simulink model "sim005"  (R2023b)
settings: Solver=FixedStepAuto  StartTime=0.0  StopTime=10.0  FixedStep=0.001  RelTol=1e-3  EnableMultiTasking=on
values from neighbouring files (symbols this model uses):
  a1 = 40    [FK.m]    (also in IK_Analytical.m = 0.04; IK_MDH.m = 0.04; IK_Position.m = 0.04; IK_Solver.m = 0.04)
  a2 = 275    [FK.m]    (also in IK_Analytical.m = 0.275; IK_MDH.m = 0.275; IK_Position.m = 0.275; IK_Solver.m = 0.275)
  a3 = 25    [FK.m]    (also in IK_Analytical.m = 0.025; IK_MDH.m = 0.025; IK_Position.m = 0.025; IK_Solver.m = 0.025)
  d1 = 342    [FK.m]    (also in IK_Analytical.m = 0.342; IK_MDH.m = 0.342; IK_Position.m = 0.342; IK_Solver.m = 0.342)
  d4 = 280    [FK.m]    (also in IK_Analytical.m = 0.28; IK_MDH.m = 0.28; IK_Position.m = 0.28; IK_Solver.m = 0.28)
  fc1 = 0    [set_mode_parameter.m]
  fc2 = 0    [set_mode_parameter.m]
  fc3 = 0    [set_mode_parameter.m]
  fc4 = 0    [set_mode_parameter.m]
  fc5 = 0    [set_mode_parameter.m]
  fc6 = 0    [set_mode_parameter.m]
  fv1 = 0    [set_mode_parameter.m]
  fv2 = 0    [set_mode_parameter.m]
  fv3 = 0    [set_mode_parameter.m]
  fv4 = 0    [set_mode_parameter.m]
  fv5 = 0    [set_mode_parameter.m]
  fv6 = 0    [set_mode_parameter.m]
  Ia1 = 0    [set_mode_parameter.m]
  Ia2 = 0    [set_mode_parameter.m]
  Ia3 = 0    [set_mode_parameter.m]
  Ia4 = 0    [set_mode_parameter.m]
  Ia5 = 0    [set_mode_parameter.m]
  Ia6 = 0    [set_mode_parameter.m]
  Ic111 = 0    [set_mode_parameter.m]
  Ic112 = 0    [set_mode_parameter.m]
  Ic113 = 0    [set_mode_parameter.m]
  Ic122 = 0    [set_mode_parameter.m]
  Ic123 = 0    [set_mode_parameter.m]
  Ic133 = 1.3676    [set_mode_parameter.m]
  Ic211 = 8.8194    [set_mode_parameter.m]
  Ic212 = 0    [set_mode_parameter.m]
  Ic213 = 0    [set_mode_parameter.m]
  Ic222 = 6.0549    [set_mode_parameter.m]
  Ic223 = 0    [set_mode_parameter.m]
  Ic233 = 0.9569    [set_mode_parameter.m]
  Ic311 = 0.0332    [set_mode_parameter.m]
  Ic312 = 0    [set_mode_parameter.m]
  Ic313 = 0    [set_mode_parameter.m]
  Ic322 = 1.8442    [set_mode_parameter.m]
  Ic323 = 0    [set_mode_parameter.m]
  Ic333 = 1.0560    (= 1.056)    [set_mode_parameter.m]
  Ic411 = 0.1448    [set_mode_parameter.m]
  Ic412 = 0    [set_mode_parameter.m]
  Ic413 = 0    [set_mode_parameter.m]
  Ic422 = 0.0015    [set_mode_parameter.m]
  Ic423 = 0    [set_mode_parameter.m]
  Ic433 = 0.0822    [set_mode_parameter.m]
  Ic511 = 0    [set_mode_parameter.m]
  Ic512 = 0    [set_mode_parameter.m]
  Ic513 = 0    [set_mode_parameter.m]
  Ic522 = 0.0121    [set_mode_parameter.m]
  Ic523 = 0    [set_mode_parameter.m]
  Ic533 = 0.0299    [set_mode_parameter.m]
  Ic611 = 0.0134    [set_mode_parameter.m]
  Ic612 = 0    [set_mode_parameter.m]
  Ic613 = 0    [set_mode_parameter.m]
  Ic622 = 0    [set_mode_parameter.m]
  Ic623 = 0    [set_mode_parameter.m]
  Ic633 = 0.0051    [set_mode_parameter.m]
  m = (c1*px + s1*py) - dt*(c1*ax + s1*ay) - a1    [IK_6DOF_Robot.m]    (also in IK_MDH.m = pwx_1 - a1; IK_MDH_Robot.m = rho - a1)
  m1 = 0.167    [set_mode_parameter.m]
  m2 = 1    [set_mode_parameter.m]
  m3 = 0.5    [set_mode_parameter.m]
  m4 = 0.333    [set_mode_parameter.m]
  m5 = 0.25    [set_mode_parameter.m]
  m6 = 0.2    [set_mode_parameter.m]
  mc11 = 0    [set_mode_parameter.m]
  mc12 = 0    [set_mode_parameter.m]
  mc13 = 0.2    [set_mode_parameter.m]
  mc21 = 0.1291    [set_mode_parameter.m]
  mc22 = 0    [set_mode_parameter.m]
  mc23 = 3.3117    [set_mode_parameter.m]
  mc31 = 1.6484    [set_mode_parameter.m]
  mc32 = 0    [set_mode_parameter.m]
  mc33 = 0.8748    [set_mode_parameter.m]
  mc41 = 0.3200    (= 0.32)    [set_mode_parameter.m]
  mc42 = 0.2324    [set_mode_parameter.m]
  mc43 = 0.7083    [set_mode_parameter.m]
  mc51 = 0.4574    [set_mode_parameter.m]
  mc52 = 0    [set_mode_parameter.m]
  mc53 = 0.6427    [set_mode_parameter.m]
  mc61 = 0.3200    (= 0.32)    [set_mode_parameter.m]
  mc62 = -0.0513    [set_mode_parameter.m]
  mc63 = 0.6417    [set_mode_parameter.m]
  N = size(waypoints, 2)    [run_trajectory.m]
  s = zc - d(1)    [inverse_kinematics_6dof.m]
  XB4 = SerialLink([L1 L2 L3 L4 L5 L6], 'name', 'XB4')    [Toolbox_Motheds_1.m]
undefined symbols (not defined in the file or in its folder): X, Y, Z
libraries: sm_lib x56, nesl_utility x31, simulink x2
(part 2 of 2)

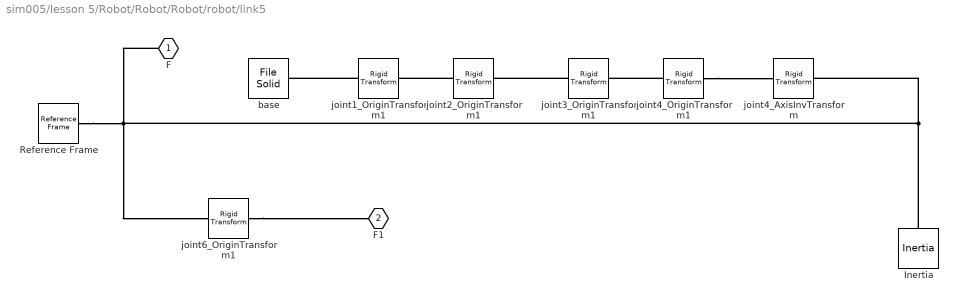
== system sim005/lesson 5/Robot/Robot/Robot/robot/link5 ==
  Inertia : sm_lib/Body Elements/Inertia  InertiaType=Custom  Mass=m5  MassUnits=kg  CenterOfMass=[mc51 mc52 mc53]  CenterOfMassUnits=m  MomentsOfInertia=[Ic511 Ic522 Ic533]  MomentsOfInertiaUnits=kg*m^2  ProductsOfInertia=[Ic523 Ic513 Ic512]  ProductsOfInertiaUnits=kg*m^2  GraphicType=Marker  MarkerShape=Inertia  MarkerSize=20  GraphicVisPropType=SimpleVisualProperties  GraphicDiffuseColor=[0.5 0.5 0.5]  GraphicSpecularColor=[0.5 0.5 0.5 1.0]  GraphicAmbientColor=[0.15 0.15 0.15 1.0]  GraphicEmissiveColor=[0.0 0.0 0.0 1.0]  GraphicShininess=75  GraphicOpacity=1.0
  Reference Frame : sm_lib/Frames and Transforms/Reference Frame
  base : sm_lib/Body Elements/File Solid  ExtGeomFileName=/home/jiehuang/Documents/Custom-Robot/Matlab_Study/Matlab2023Project/XB4-Robot/Mode/XB4-5.STL  UnitType=Custom  ExtGeomFileUnits=mm  StepReaderType=HEX  ExportConvexHullGeometry=off  InertiaType=Custom  Mass=0  MassUnits=kg  CenterOfMass=[0 0 0]  CenterOfMassUnits=m  MomentsOfInertia=[0 0 0]  MomentsOfInertiaUnits=kg*m^2  ProductsOfInertia=[0 0 0]  ProductsOfInertiaUnits=kg*m^2  BasedOnType=Density  Density=1000  DensityUnits=kg/(m^3)  DoExposeReferenceFrame=on  SerializedFrames=<Frames/>  GraphicType=FromGeometry  MarkerShape=Sphere  MarkerSize=10  GraphicVisPropType=SimpleVisualProperties  GraphicDiffuseColor=[0.5 0.5 0.5]  GraphicSpecularColor=[0.5 0.5 0.5 1.0]  GraphicAmbientColor=[0.15 0.15 0.15 1.0]  GraphicEmissiveColor=[0.0 0.0 0.0 1.0]  GraphicShininess=75  GraphicOpacity=1.0
  joint1_OriginTransform1 : sm_lib/Frames and Transforms/Rigid Transform  TranslationMethod=Cartesian  TranslationStandardOffset=0  TranslationStandardOffsetUnits=m  TranslationStandardAxis=+Z  TranslationCartesianOffset=[0 0 d1]  TranslationCartesianOffsetUnits=m  TranslationROffset=0  TranslationROffsetUnits=m  TranslationZOffset=0  TranslationZOffsetUnits=m  TranslationThetaOffset=0  TranslationThetaOffsetUnits=deg  RotationMethod=RotationSequence  RotationAngleUnits=deg  RotationStandardAxis=+Z  RotationAngle=0.0  RotationArbitraryAxis=[0 0 1]  FollAlignAxisA=+X  BaseAlignAxisA=+Y  FollAlignAxisB=+Y  BaseAlignAxisB=+Z  RotationSequenceAxes=BaseAxes  RotationSequence=XYZ  RotationSequenceAngles=[0 0 0]  RotationSequenceAnglesUnits=rad  RotationMatrix=[1 0 0; 0 1 0; 0 0 1]  Quaternion=[1 0 0 0]
  joint2_OriginTransform1 : sm_lib/Frames and Transforms/Rigid Transform  TranslationMethod=Cartesian  TranslationStandardOffset=0  TranslationStandardOffsetUnits=m  TranslationStandardAxis=+Z  TranslationCartesianOffset=[a1 0 0]  TranslationCartesianOffsetUnits=m  TranslationROffset=0  TranslationROffsetUnits=m  TranslationZOffset=0  TranslationZOffsetUnits=m  TranslationThetaOffset=0  TranslationThetaOffsetUnits=deg  RotationMethod=RotationSequence  RotationAngleUnits=deg  RotationStandardAxis=+Z  RotationAngle=0.0  RotationArbitraryAxis=[0 0 1]  FollAlignAxisA=+X  BaseAlignAxisA=+Y  FollAlignAxisB=+Y  BaseAlignAxisB=+Z  RotationSequenceAxes=FollowerAxes  RotationSequence=XYZ  RotationSequenceAngles=[-pi/2 0 -pi/2]  RotationSequenceAnglesUnits=rad  RotationMatrix=[1 0 0; 0 1 0; 0 0 1]  Quaternion=[1 0 0 0]
  joint3_OriginTransform1 : sm_lib/Frames and Transforms/Rigid Transform  TranslationMethod=Cartesian  TranslationStandardOffset=0  TranslationStandardOffsetUnits=m  TranslationStandardAxis=+Z  TranslationCartesianOffset=[a2 0 0]  TranslationCartesianOffsetUnits=m  TranslationROffset=0  TranslationROffsetUnits=m  TranslationZOffset=0  TranslationZOffsetUnits=m  TranslationThetaOffset=0  TranslationThetaOffsetUnits=deg  RotationMethod=RotationSequence  RotationAngleUnits=deg  RotationStandardAxis=+Z  RotationAngle=0.0  RotationArbitraryAxis=[0 0 1]  FollAlignAxisA=+X  BaseAlignAxisA=+Y  FollAlignAxisB=+Y  BaseAlignAxisB=+Z  RotationSequenceAxes=FollowerAxes  RotationSequence=XYZ  RotationSequenceAngles=[0 0 0]  RotationSequenceAnglesUnits=rad  RotationMatrix=[1 0 0; 0 1 0; 0 0 1]  Quaternion=[1 0 0 0]
  joint4_AxisInvTransform : sm_lib/Frames and Transforms/Rigid Transform  TranslationMethod=Cartesian  TranslationStandardOffset=0  TranslationStandardOffsetUnits=m  TranslationStandardAxis=+Z  TranslationCartesianOffset=[0 0 0]  TranslationCartesianOffsetUnits=m  TranslationROffset=0  TranslationROffsetUnits=m  TranslationZOffset=0  TranslationZOffsetUnits=m  TranslationThetaOffset=0  TranslationThetaOffsetUnits=deg  RotationMethod=RotationSequence  RotationAngleUnits=rad  RotationStandardAxis=+Z  RotationAngle=1.570796  RotationArbitraryAxis=[0 1 0]  FollAlignAxisA=+X  BaseAlignAxisA=+Y  FollAlignAxisB=+Y  BaseAlignAxisB=+Z  RotationSequenceAxes=FollowerAxes  RotationSequence=XYZ  RotationSequenceAngles=[pi/2 0 0]  RotationSequenceAnglesUnits=rad  RotationMatrix=[1 0 0; 0 1 0; 0 0 1]  Quaternion=[1 0 0 0]
  joint4_OriginTransform1 : sm_lib/Frames and Transforms/Rigid Transform  TranslationMethod=Cartesian  TranslationStandardOffset=0  TranslationStandardOffsetUnits=m  TranslationStandardAxis=+Z  TranslationCartesianOffset=[a3 d4 0]  TranslationCartesianOffsetUnits=m  TranslationROffset=0  TranslationROffsetUnits=m  TranslationZOffset=0  TranslationZOffsetUnits=m  TranslationThetaOffset=0  TranslationThetaOffsetUnits=deg  RotationMethod=RotationSequence  RotationAngleUnits=deg  RotationStandardAxis=+Z  RotationAngle=0.0  RotationArbitraryAxis=[0 0 1]  FollAlignAxisA=+X  BaseAlignAxisA=+Y  FollAlignAxisB=+Y  BaseAlignAxisB=+Z  RotationSequenceAxes=FollowerAxes  RotationSequence=XYZ  RotationSequenceAngles=[-pi/2 0 0]  RotationSequenceAnglesUnits=rad  RotationMatrix=[1 0 0; 0 1 0; 0 0 1]  Quaternion=[1 0 0 0]
  joint6_OriginTransform1 : sm_lib/Frames and Transforms/Rigid Transform  TranslationMethod=Cartesian  TranslationStandardOffset=0  TranslationStandardOffsetUnits=m  TranslationStandardAxis=+Z  TranslationCartesianOffset=[0 0 0]  TranslationCartesianOffsetUnits=m  TranslationROffset=0  TranslationROffsetUnits=m  TranslationZOffset=0  TranslationZOffsetUnits=m  TranslationThetaOffset=0  TranslationThetaOffsetUnits=deg  RotationMethod=RotationSequence  RotationAngleUnits=deg  RotationStandardAxis=+Z  RotationAngle=0.0  RotationArbitraryAxis=[0 0 1]  FollAlignAxisA=+X  BaseAlignAxisA=+Y  FollAlignAxisB=+Y  BaseAlignAxisB=+Z  RotationSequenceAxes=FollowerAxes  RotationSequence=XYZ  RotationSequenceAngles=[-pi/2 0 0]  RotationSequenceAnglesUnits=rad  RotationMatrix=[1 0 0; 0 1 0; 0 0 1]  Quaternion=[1 0 0 0]
  F : PMIOPort  Side=Left
  F1 : PMIOPort  Port=2  Side=Right
  connections:
  Reference Frame/RConn1 -- Inertia/RConn1 -- joint4_AxisInvTransform/RConn1 -- F/RConn1 -- joint6_OriginTransform1/LConn1
  joint6_OriginTransform1/RConn1 -- F1/RConn1
  joint1_OriginTransform1/LConn1 -- base/RConn1
  joint3_OriginTransform1/LConn1 -- joint2_OriginTransform1/RConn1
  joint4_OriginTransform1/LConn1 -- joint3_OriginTransform1/RConn1
  joint2_OriginTransform1/LConn1 -- joint1_OriginTransform1/RConn1
  joint4_OriginTransform1/RConn1 -- joint4_AxisInvTransform/LConn1

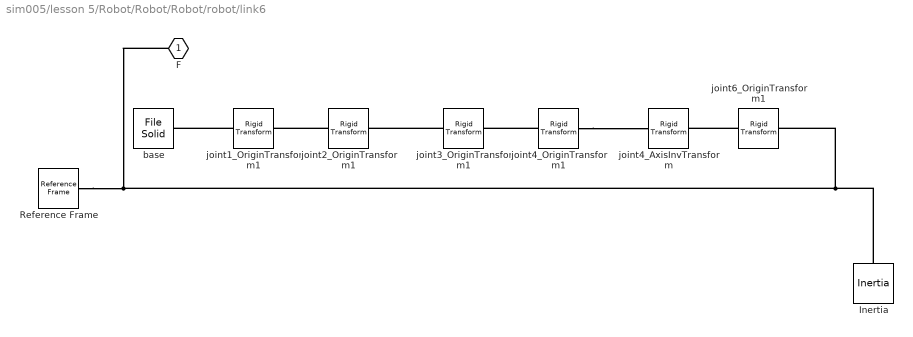
== system sim005/lesson 5/Robot/Robot/Robot/robot/link6 ==
  Inertia : sm_lib/Body Elements/Inertia  InertiaType=Custom  Mass=m6  MassUnits=kg  CenterOfMass=[mc61 mc62 mc63]  CenterOfMassUnits=m  MomentsOfInertia=[Ic611 Ic622 Ic633 ]  MomentsOfInertiaUnits=kg*m^2  ProductsOfInertia=[Ic623 Ic613 Ic612]  ProductsOfInertiaUnits=kg*m^2  GraphicType=Marker  MarkerShape=Inertia  MarkerSize=20  GraphicVisPropType=SimpleVisualProperties  GraphicDiffuseColor=[0.5 0.5 0.5]  GraphicSpecularColor=[0.5 0.5 0.5 1.0]  GraphicAmbientColor=[0.15 0.15 0.15 1.0]  GraphicEmissiveColor=[0.0 0.0 0.0 1.0]  GraphicShininess=75  GraphicOpacity=1.0
  Reference Frame : sm_lib/Frames and Transforms/Reference Frame
  base : sm_lib/Body Elements/File Solid  ExtGeomFileName=/home/jiehuang/Documents/Custom-Robot/Matlab_Study/Matlab2023Project/XB4-Robot/Mode/XB4-6.STL  UnitType=Custom  ExtGeomFileUnits=mm  StepReaderType=HEX  ExportConvexHullGeometry=off  InertiaType=Custom  Mass=0  MassUnits=kg  CenterOfMass=[0 0 0]  CenterOfMassUnits=m  MomentsOfInertia=[0 0 0]  MomentsOfInertiaUnits=kg*m^2  ProductsOfInertia=[0 0 0]  ProductsOfInertiaUnits=kg*m^2  BasedOnType=Density  Density=1000  DensityUnits=kg/(m^3)  DoExposeReferenceFrame=on  SerializedFrames=<Frames/>  GraphicType=FromGeometry  MarkerShape=Sphere  MarkerSize=10  GraphicVisPropType=SimpleVisualProperties  GraphicDiffuseColor=[0.5 0.5 0.5]  GraphicSpecularColor=[0.5 0.5 0.5 1.0]  GraphicAmbientColor=[0.15 0.15 0.15 1.0]  GraphicEmissiveColor=[0.0 0.0 0.0 1.0]  GraphicShininess=75  GraphicOpacity=1.0
  joint1_OriginTransform1 : sm_lib/Frames and Transforms/Rigid Transform  TranslationMethod=Cartesian  TranslationStandardOffset=0  TranslationStandardOffsetUnits=m  TranslationStandardAxis=+Z  TranslationCartesianOffset=[0 0 d1]  TranslationCartesianOffsetUnits=m  TranslationROffset=0  TranslationROffsetUnits=m  TranslationZOffset=0  TranslationZOffsetUnits=m  TranslationThetaOffset=0  TranslationThetaOffsetUnits=deg  RotationMethod=RotationSequence  RotationAngleUnits=deg  RotationStandardAxis=+Z  RotationAngle=0.0  RotationArbitraryAxis=[0 0 1]  FollAlignAxisA=+X  BaseAlignAxisA=+Y  FollAlignAxisB=+Y  BaseAlignAxisB=+Z  RotationSequenceAxes=BaseAxes  RotationSequence=XYZ  RotationSequenceAngles=[0 0 0]  RotationSequenceAnglesUnits=rad  RotationMatrix=[1 0 0; 0 1 0; 0 0 1]  Quaternion=[1 0 0 0]
  joint2_OriginTransform1 : sm_lib/Frames and Transforms/Rigid Transform  TranslationMethod=Cartesian  TranslationStandardOffset=0  TranslationStandardOffsetUnits=m  TranslationStandardAxis=+Z  TranslationCartesianOffset=[a1 0 0]  TranslationCartesianOffsetUnits=m  TranslationROffset=0  TranslationROffsetUnits=m  TranslationZOffset=0  TranslationZOffsetUnits=m  TranslationThetaOffset=0  TranslationThetaOffsetUnits=deg  RotationMethod=RotationSequence  RotationAngleUnits=deg  RotationStandardAxis=+Z  RotationAngle=0.0  RotationArbitraryAxis=[0 0 1]  FollAlignAxisA=+X  BaseAlignAxisA=+Y  FollAlignAxisB=+Y  BaseAlignAxisB=+Z  RotationSequenceAxes=FollowerAxes  RotationSequence=XYZ  RotationSequenceAngles=[-pi/2 0 -pi/2]  RotationSequenceAnglesUnits=rad  RotationMatrix=[1 0 0; 0 1 0; 0 0 1]  Quaternion=[1 0 0 0]
  joint3_OriginTransform1 : sm_lib/Frames and Transforms/Rigid Transform  TranslationMethod=Cartesian  TranslationStandardOffset=0  TranslationStandardOffsetUnits=m  TranslationStandardAxis=+Z  TranslationCartesianOffset=[a2 0 0]  TranslationCartesianOffsetUnits=m  TranslationROffset=0  TranslationROffsetUnits=m  TranslationZOffset=0  TranslationZOffsetUnits=m  TranslationThetaOffset=0  TranslationThetaOffsetUnits=deg  RotationMethod=RotationSequence  RotationAngleUnits=deg  RotationStandardAxis=+Z  RotationAngle=0.0  RotationArbitraryAxis=[0 0 1]  FollAlignAxisA=+X  BaseAlignAxisA=+Y  FollAlignAxisB=+Y  BaseAlignAxisB=+Z  RotationSequenceAxes=FollowerAxes  RotationSequence=XYZ  RotationSequenceAngles=[0 0 0]  RotationSequenceAnglesUnits=rad  RotationMatrix=[1 0 0; 0 1 0; 0 0 1]  Quaternion=[1 0 0 0]
  joint4_AxisInvTransform : sm_lib/Frames and Transforms/Rigid Transform  TranslationMethod=Cartesian  TranslationStandardOffset=0  TranslationStandardOffsetUnits=m  TranslationStandardAxis=+Z  TranslationCartesianOffset=[0 0 0]  TranslationCartesianOffsetUnits=m  TranslationROffset=0  TranslationROffsetUnits=m  TranslationZOffset=0  TranslationZOffsetUnits=m  TranslationThetaOffset=0  TranslationThetaOffsetUnits=deg  RotationMethod=RotationSequence  RotationAngleUnits=rad  RotationStandardAxis=+Z  RotationAngle=1.570796  RotationArbitraryAxis=[0 1 0]  FollAlignAxisA=+X  BaseAlignAxisA=+Y  FollAlignAxisB=+Y  BaseAlignAxisB=+Z  RotationSequenceAxes=FollowerAxes  RotationSequence=XYZ  RotationSequenceAngles=[pi/2 0 0]  RotationSequenceAnglesUnits=rad  RotationMatrix=[1 0 0; 0 1 0; 0 0 1]  Quaternion=[1 0 0 0]
  joint4_OriginTransform1 : sm_lib/Frames and Transforms/Rigid Transform  TranslationMethod=Cartesian  TranslationStandardOffset=0  TranslationStandardOffsetUnits=m  TranslationStandardAxis=+Z  TranslationCartesianOffset=[a3 d4 0]  TranslationCartesianOffsetUnits=m  TranslationROffset=0  TranslationROffsetUnits=m  TranslationZOffset=0  TranslationZOffsetUnits=m  TranslationThetaOffset=0  TranslationThetaOffsetUnits=deg  RotationMethod=RotationSequence  RotationAngleUnits=deg  RotationStandardAxis=+Z  RotationAngle=0.0  RotationArbitraryAxis=[0 0 1]  FollAlignAxisA=+X  BaseAlignAxisA=+Y  FollAlignAxisB=+Y  BaseAlignAxisB=+Z  RotationSequenceAxes=FollowerAxes  RotationSequence=XYZ  RotationSequenceAngles=[-pi/2 0 0]  RotationSequenceAnglesUnits=rad  RotationMatrix=[1 0 0; 0 1 0; 0 0 1]  Quaternion=[1 0 0 0]
  joint6_OriginTransform1 : sm_lib/Frames and Transforms/Rigid Transform  TranslationMethod=Cartesian  TranslationStandardOffset=0  TranslationStandardOffsetUnits=m  TranslationStandardAxis=+Z  TranslationCartesianOffset=[0 0 0]  TranslationCartesianOffsetUnits=m  TranslationROffset=0  TranslationROffsetUnits=m  TranslationZOffset=0  TranslationZOffsetUnits=m  TranslationThetaOffset=0  TranslationThetaOffsetUnits=deg  RotationMethod=RotationSequence  RotationAngleUnits=deg  RotationStandardAxis=+Z  RotationAngle=0.0  RotationArbitraryAxis=[0 0 1]  FollAlignAxisA=+X  BaseAlignAxisA=+Y  FollAlignAxisB=+Y  BaseAlignAxisB=+Z  RotationSequenceAxes=FollowerAxes  RotationSequence=XYZ  RotationSequenceAngles=[-pi/2 0 0]  RotationSequenceAnglesUnits=rad  RotationMatrix=[1 0 0; 0 1 0; 0 0 1]  Quaternion=[1 0 0 0]
  F : PMIOPort  Side=Left
  connections:
  Reference Frame/RConn1 -- joint6_OriginTransform1/RConn1 -- Inertia/RConn1 -- F/RConn1
  joint6_OriginTransform1/LConn1 -- joint4_AxisInvTransform/RConn1
  joint1_OriginTransform1/LConn1 -- base/RConn1
  joint3_OriginTransform1/LConn1 -- joint2_OriginTransform1/RConn1
  joint4_OriginTransform1/RConn1 -- joint4_AxisInvTransform/LConn1
  joint4_OriginTransform1/LConn1 -- joint3_OriginTransform1/RConn1
  joint2_OriginTransform1/LConn1 -- joint1_OriginTransform1/RConn1

== matlab function sim005/lesson 5/Subsystem/三阶曲线规划/三关节/Interpolation3 ==
  data: state output; Enable input; Y output; plan3_A input; tf input; t input
function [state, Y]  = Interpolate3(Enable,plan3_A,tf,t)
%% input
a0 = plan3_A(1);
a1 = plan3_A(2);
a2 = plan3_A(3);
a3 = plan3_A(4);
Y = 0;
%% output
if Enable == 1
    if t <=tf
    Y = a0 + a1*t + a2*t^2 + a3*t^3; 
    state =1;
    else
    Y = a0 + a1*tf + a2*tf^2 + a3*tf^3;
    state = 1;
    end
else 
    Y = 0;
    state = 0;
end
end

== matlab function sim005/lesson 5/Subsystem/三阶曲线规划/二关节/3_planning1 ==
  data: state output; plan3_A output; g_vs parameter; g_ve parameter; S input; tf input; tf output
function [state, plan3_A,tf] =planning3( g_vs, g_ve,S,tf)
% 三次多项式算法主程序
% vs初始速度m/min,ve末速度m/min,S总位移m,
% 基础插补规划函数
% 三次多项式速度规划
    a0 = 0 ;
    a1 = g_vs ;
    a2 = 3*S/tf^2 - 2* g_vs/tf - g_ve/tf;
    a3 = -2*S/tf^3 - (g_vs+g_ve)/tf^2;
    state = 1;
    plan3_A = [a0 a1 a2 a3];
    tf =tf ;

end

== matlab function sim005/lesson 5/Subsystem/三阶曲线规划/二关节/Interpolation3 ==
  data: state output; Enable input; Y output; plan3_A input; tf input; t input
function [state, Y]  = Interpolate3(Enable,plan3_A,tf,t)
%% input
a0 = plan3_A(1);
a1 = plan3_A(2);
a2 = plan3_A(3);
a3 = plan3_A(4);
Y = 0;
%% output
if Enable == 1
    if t <=tf
    Y = a0 + a1*t + a2*t^2 + a3*t^3; 
    state =1;
    else
    Y = a0 + a1*tf + a2*tf^2 + a3*tf^3;
    state = 1;
    end
else 
    Y = 0;
    state = 0;
end
end

== matlab function sim005/lesson 5/Subsystem/三阶曲线规划/五关节/3_planning1 ==
  data: state output; plan3_A output; g_vs parameter; g_ve parameter; S input; tf input; tf output
function [state, plan3_A,tf] =planning3( g_vs, g_ve,S,tf)
% 三次多项式算法主程序
% vs初始速度m/min,ve末速度m/min,S总位移m,
% 基础插补规划函数
% 三次多项式速度规划
    a0 = 0 ;
    a1 = g_vs ;
    a2 = 3*S/tf^2 - 2* g_vs/tf - g_ve/tf;
    a3 = -2*S/tf^3 - (g_vs+g_ve)/tf^2;
    state = 1;
    plan3_A = [a0 a1 a2 a3];
    tf =tf ;

end

== matlab function sim005/lesson 5/Subsystem/三阶曲线规划/五关节/Interpolation3 ==
  data: state output; Enable input; Y output; plan3_A input; tf input; t input
function [state, Y]  = Interpolate3(Enable,plan3_A,tf,t)
%% input
a0 = plan3_A(1);
a1 = plan3_A(2);
a2 = plan3_A(3);
a3 = plan3_A(4);
Y = 0;
%% output
if Enable == 1
    if t <=tf
    Y = a0 + a1*t + a2*t^2 + a3*t^3; 
    state =1;
    else
    Y = a0 + a1*tf + a2*tf^2 + a3*tf^3;
    state = 1;
    end
else 
    Y = 0;
    state = 0;
end
end

== matlab function sim005/lesson 5/Subsystem/三阶曲线规划/六关节/3_planning1 ==
  data: state output; plan3_A output; g_vs parameter; g_ve parameter; S input; tf input; tf output
function [state, plan3_A,tf] =planning3( g_vs, g_ve,S,tf)
% 三次多项式算法主程序
% vs初始速度m/min,ve末速度m/min,S总位移m,
% 基础插补规划函数
% 三次多项式速度规划
    a0 = 0 ;
    a1 = g_vs ;
    a2 = 3*S/tf^2 - 2* g_vs/tf - g_ve/tf;
    a3 = -2*S/tf^3 - (g_vs+g_ve)/tf^2;
    state = 1;
    plan3_A = [a0 a1 a2 a3];
    tf =tf ;

end

== matlab function sim005/lesson 5/Subsystem/三阶曲线规划/六关节/Interpolation3 ==
  data: state output; Enable input; Y output; plan3_A input; tf input; t input
function [state, Y]  = Interpolate3(Enable,plan3_A,tf,t)
%% input
a0 = plan3_A(1);
a1 = plan3_A(2);
a2 = plan3_A(3);
a3 = plan3_A(4);
Y = 0;
%% output
if Enable == 1
    if t <=tf
    Y = a0 + a1*t + a2*t^2 + a3*t^3; 
    state =1;
    else
    Y = a0 + a1*tf + a2*tf^2 + a3*tf^3;
    state = 1;
    end
else 
    Y = 0;
    state = 0;
end
end

== matlab function sim005/lesson 5/Subsystem/三阶曲线规划/四关节/3_planning1 ==
  data: state output; plan3_A output; g_vs parameter; g_ve parameter; S input; tf input; tf output
function [state, plan3_A,tf] =planning3( g_vs, g_ve,S,tf)
% 三次多项式算法主程序
% vs初始速度m/min,ve末速度m/min,S总位移m,
% 基础插补规划函数
% 三次多项式速度规划
    a0 = 0 ;
    a1 = g_vs ;
    a2 = 3*S/tf^2 - 2* g_vs/tf - g_ve/tf;
    a3 = -2*S/tf^3 - (g_vs+g_ve)/tf^2;
    state = 1;
    plan3_A = [a0 a1 a2 a3];
    tf =tf ;

end

== matlab function sim005/lesson 5/Subsystem/三阶曲线规划/四关节/Interpolation3 ==
  data: state output; Enable input; Y output; plan3_A input; tf input; t input
function [state, Y]  = Interpolate3(Enable,plan3_A,tf,t)
%% input
a0 = plan3_A(1);
a1 = plan3_A(2);
a2 = plan3_A(3);
a3 = plan3_A(4);
Y = 0;
%% output
if Enable == 1
    if t <=tf
    Y = a0 + a1*t + a2*t^2 + a3*t^3; 
    state =1;
    else
    Y = a0 + a1*tf + a2*tf^2 + a3*tf^3;
    state = 1;
    end
else 
    Y = 0;
    state = 0;
end
end

== matlab function sim005/lesson 5/DH-CC1 ==
  data: KPS44 input; KPS6 output
function KPS6 = FK(KPS44)

%% 输入 KPS44：4×4 齐次变换矩阵
% 位置
px = KPS44(1,4);
py = KPS44(2,4);
pz = KPS44(3,4);

%% 姿态（从旋转矩阵中提取 RPY）
R = KPS44(1:3, 1:3);

r11 = R(1,1); r12 = R(1,2); r13 = R(1,3);
r21 = R(2,1); r22 = R(2,2); r23 = R(2,3);
r31 = R(3,1); r32 = R(3,2); r33 = R(3,3);

%% Pitch 可能引起奇异，因此加 eps
eps = 1e-9;

%% Roll-Pitch-Yaw (X-Y-Z 欧拉角)
roll  = atan2(r32, r33); 
pitch = atan2(-r31, sqrt(r32^2 + r33^2 + eps)); 
yaw   = atan2(r21, r11);

%% 输出 1×6 
KPS6 = [px, py, pz, roll, pitch, yaw];

end

== matlab function sim005/lesson 5/DH1 ==
  data: Radian input; KPS44 output
function KPS44 = FK(Radian)

%% 输入关节角（单位 rad）
theta1 = Radian(1);
theta2 = Radian(2);
theta3 = Radian(3);
theta4 = Radian(4);
theta5 = Radian(5);
theta6 = Radian(6);

%% -------- 1. Modified DH 参数 --------
d1 = 342; 
a1 = 40;  alpha1 = -pi/2;

d2 = 0;   
a2 = 275; alpha2 = 0;

d3 = 0;   
a3 = 25;  alpha3 = -pi/2;

d4 = 280; 
a4 = 0;   alpha4 = pi/2;

d5 = 0;   
a5 = 0;   alpha5 = -pi/2;

dt = 73;
d6 = dt;  
a6 = 0;   alpha6 = 0;

%% -------- 2. 建立 DH 变换函数 --------
DH = @(a,alpha,d,theta) [ ...
    cos(theta)            -sin(theta)             0              a;
    sin(theta)*cos(alpha) cos(theta)*cos(alpha)  -sin(alpha)  -sin(alpha)*d;
    sin(theta)*sin(alpha) cos(theta)*sin(alpha)   cos(alpha)   cos(alpha)*d;
    0                     0                       0              1 ];

%% -------- 3. 计算 T1 ~ T6 --------
T1 = DH(a1,alpha1,d1,theta1);
T2 = DH(a2,alpha2,d2,theta2);
T3 = DH(a3,alpha3,d3,theta3);
T4 = DH(a4,alpha4,d4,theta4);
T5 = DH(a5,alpha5,d5,theta5);
T6 = DH(a6,alpha6,d6,theta6);

%% -------- 4. Base 与 Tool 变换矩阵（教材给的）--------
Tbase = [1 0 0 0;
         0 1 0 0;
         0 0 1 0;
         0 0 0 1];

Ttool = [1 0 0 0;
         0 1 0 0;
         0 0 1 0;
         0 0 0 1];

%% -------- 5. 输出机器人末端位姿 --------
KPS44 = Tbase * T1 * T2 * T3 * T4 * T5 * T6 * Ttool;

end

== matlab function sim005/lesson 5/DH-IK ==
  data: KPS44 input; Radian output; RAngle input
function Radian = IK(KPS44, RAngle)
%% ===== 固定输出大小 =====
Radian = zeros(6,1);

%% ===== 参数定义 =====
d1 = 342; a1 = 40; a2 = 275; a3 = 25; d4 = 280; d6 = 73;

%% ===== Base 与 Tool 转换 =====
Tbase = [1 0 0 0; 0 1 0 0; 0 0 1 d1; 0 0 0 1];
Ttool = [1 0 0 0; 0 1 0 0; 0 0 1 d6; 0 0 0 1];

R44 = inv(Tbase) * KPS44 * inv(Ttool);

%% ===== 末端姿态分解 =====
x  = R44(1,4);
y  = R44(2,4);
z  = R44(3,4);

nx = R44(1,1); ny = R44(2,1); nz = R44(3,1);
ox = R44(1,2); oy = R44(2,2); oz = R44(3,2);
ax = R44(1,3); ay = R44(2,3); az = R44(3,3);

%% =====================================
%   1) θ1
%% =====================================
Q1 = zeros(1,2);
L = sqrt(x^2 + y^2 - d4^2);

Q1(1) = atan2(y, x) - atan2(d4,  L);
Q1(2) = atan2(y, x) - atan2(d4, -L);

%% =====================================
%   2) θ3
%% =====================================
Q3 = zeros(1,4);
k = 1;

for i = 1:2
    th1 = Q1(i);
    c1 = cos(th1); s1 = sin(th1);

    K = x*c1 + y*s1 - a1;
    D = (K^2 + (z-d1)^2 - a2^2 - a3^2) / (2*a2*a3);

    if abs(D) <= 1
        Q3(k)   = atan2( sqrt(1-D^2), D );
        Q3(k+1) = atan2(-sqrt(1-D^2), D );
    else
        Q3(k)   = 0;
        Q3(k+1) = 0;
    end

    k = k + 2;
end

%% =====================================
%   3) θ2
%% =====================================
Q2 = zeros(1,4);
k = 1;

for i = 1:2
    th1 = Q1(i);
    c1 = cos(th1); s1 = sin(th1);

    for j = 1:2
        th3 = Q3((i-1)*2 + j);
        c3 = cos(th3); s3 = sin(th3);

        A = a2 + a3*c3;
        B = a3*s3;

        K = x*c1 + y*s1 - a1;

        Q2(k) = atan2(z - d1, K) - atan2(B, A);

        k = k + 1;
    end
end

%% =====================================
%   4) 求 θ4 θ5 θ6
%% =====================================
QQ = zeros(8,6);
row = 1;

for i = 1:4
    th1 = Q1( ceil(i/2) );
    th2 = Q2(i);
    th3 = Q3(i);

    c1=cos(th1); s1=sin(th1);
    c2=cos(th2); s2=sin(th2);
    c3=cos(th3); s3=sin(th3);

    R03 = [
        c1*c2*c3-c1*s2*s3, -c1*c2*s3-c1*s2*c3, c1*s2;
        s1*c2*c3-s1*s2*s3, -s1*c2*s3-s1*s2*c3, s1*s2;
        s2*c3+c2*s3,       -s2*s3+c2*c3,      -c2 ];

    R36 = R03' * [nx ox ax; ny oy ay; nz oz az];

    th5 = atan2( sqrt( R36(1,3)^2 + R36(2,3)^2 ), R36(3,3) );
    th4 = atan2( R36(2,3), R36(1,3) );
    th6 = atan2( R36(3,2), -R36(3,1) );

    QQ(row,:) = [th1 th2 th3 th4 th5 th6];
    QQ(row+4,:) = [th1 th2 th3 th4 -th5 th6+pi];

    row = row + 1;
end

%% =====================================
%   5) 选择最优解（与当前角度最接近）
%% =====================================
bestIndex = 1;
bestVal = inf;

for i = 1:8
    diff = sum(abs(QQ(i,:)' - RAngle));
    if diff < bestVal
        bestVal = diff;
        bestIndex = i;
    end
end

Radian = QQ(bestIndex,:)';

end

== matlab function sim005/lesson 5/DH-IK-CC ==
  data: KPS6 input; KPS44 output
function KPS44  = IK(KPS6)
%% input 
x = KPS6(1);
y = KPS6(2);
z = KPS6(3);
p = KPS6(4);
q = KPS6(5);
r = KPS6(6);

%% output
KPS44 = eye(4);

%% RPY→旋转矩阵
sx = sin(p); cx = cos(p);
sy = sin(q); cy = cos(q);
sz = sin(r); cz = cos(r);

% R = Rz(r)*Ry(q)*Rx(p)
KPS44(1,1) = cy*cz;
KPS44(1,2) = -cy*sz;
KPS44(1,3) = sy;

KPS44(2,1) = cx*sz + cz*sx*sy;
KPS44(2,2) = cx*cz - sx*sy*sz;
KPS44(2,3) = -cy*sx;

KPS44(3,1) = sx*sz - cx*cz*sy;
KPS44(3,2) = cz*sx + cx*sy*sz;
KPS44(3,3) = cx*cy;

%% 位置
KPS44(1,4) = x;
KPS44(2,4) = y;
KPS44(3,4) = z;

end

== matlab function sim005/lesson 5/Robot/Robot/Robot/robot/Jm ==
  data: u input; y output; Jm input
function y = fcn(u,Jm)
%#codegen

% Jm=[200; 250; 150; 100; 50; 20];%关节惯性
y = Jm.*u;
end

== matlab function sim005/lesson 5/Robot/Robot/Robot/robot/friction ==
  data: u input; y output; fv input; fc input
function y = fcn(u,fv,fc)
%#codegen


% fv1=100; fc1=80; fv2=150; fc2=100; fv3=100; fc3=50; fv4=80; fc4=80; fv5=50; fc5=30; fv6=30; fc6=10;
fv1=fv(1); fc1=fc(1); fv2=fv(2); fc2=fc(2); fv3=fv(3); fc3=fc(3); fv4=fv(4); fc4=fc(4); fv5=fv(5); fc5=fc(5); fv6=fv(6); fc6=fc(6);
y=[0;0;0;0;0;0];
y(1)=(fv1*u(1)+fc1*sign(u(1)));
y(2)=(fv2*u(2)+fc2*sign(u(2)));
y(3)=(fv3*u(3)+fc3*sign(u(3)));
y(4)=(fv4*u(4)+fc4*sign(u(4)));
y(5)=(fv5*u(5)+fc5*sign(u(5)));
y(6)=(fv6*u(6)+fc6*sign(u(6)));

end

== matlab function sim005/lesson 5/Subsystem/三阶曲线规划/一关节/3_planning1 ==
  data: state output; plan3_A output; g_vs parameter; g_ve parameter; S input; tf input; tf output
function [state, plan3_A,tf] =planning3( g_vs, g_ve,S,tf)
% 三次多项式算法主程序
% vs初始速度m/min,ve末速度m/min,S总位移m,
% 基础插补规划函数
% 三次多项式速度规划
    a0 = 0 ;
    a1 = g_vs ;
    a2 = 3*S/tf^2 - 2* g_vs/tf - g_ve/tf;
    a3 = -2*S/tf^3 - (g_vs+g_ve)/tf^2;
    state = 1;
    plan3_A = [a0 a1 a2 a3];
    tf =tf ;

end

== matlab function sim005/lesson 5/Subsystem/三阶曲线规划/一关节/Interpolation3 ==
  data: state output; Enable input; Y output; plan3_A input; tf input; t input
function [state, Y]  = Interpolate3(Enable,plan3_A,tf,t)
%% input
a0 = plan3_A(1);
a1 = plan3_A(2);
a2 = plan3_A(3);
a3 = plan3_A(4);
Y = 0;
%% output
if Enable == 1
    if t <=tf
    Y = a0 + a1*t + a2*t^2 + a3*t^3; 
    state =1;
    else
    Y = a0 + a1*tf + a2*tf^2 + a3*tf^3;
    state = 1;
    end
else 
    Y = 0;
    state = 0;
end
end

== matlab function sim005/lesson 5/Subsystem/三阶曲线规划/三关节/3_planning1 ==
  data: state output; plan3_A output; g_vs parameter; g_ve parameter; S input; tf input; tf output
function [state, plan3_A,tf] =planning3( g_vs, g_ve,S,tf)
% 三次多项式算法主程序
% vs初始速度m/min,ve末速度m/min,S总位移m,
% 基础插补规划函数
% 三次多项式速度规划
    a0 = 0 ;
    a1 = g_vs ;
    a2 = 3*S/tf^2 - 2* g_vs/tf - g_ve/tf;
    a3 = -2*S/tf^3 - (g_vs+g_ve)/tf^2;
    state = 1;
    plan3_A = [a0 a1 a2 a3];
    tf =tf ;

end
